simulink model "AFMss_"  (R2016b)
settings: Solver=ode4  StartTime=0.0  StopTime=trun  FixedStep=Ts  RelTol=1e-5  EnableMultiTasking=on
PreLoadFcn:
  | VSS_CONTROL_MODE=1;
  | VSS_LINEAR_CONTROL=Simulink.Variant('VSS_CONTROL_MODE==1');
  | VSS_MPC_CONTROL=Simulink.Variant('VSS_CONTROL_MODE == 2');
  | 
  | 
  | VSS_STATE_DIRECT=Simulink.Variant('VSS_STATE_MODE==1');
  | VSS_STATE_OBS=Simulink.Variant('VSS_STATE_MODE==2');
  | VSS_STATE_DIST_OBS=Simulink.Variant('VSS_STATE_MODE==3');
  | VSS_STATE_MODE=1;
values from neighbouring files (symbols this model uses):
  dist = 1    [explore_ss_loops_distest.m]    (also in explore_ss_loops_distest_AFM.m = 0; explore_ss_loops_distest_delta.m = 0)
  K_lqr = dlqr(sys.a, sys.b, Q, R, S)    [explore_ss_loops_distest.m]    (also in explore_ss_loops_distest_AFM.m; explore_ss_loops_distest_delta.m = dlqr(sys_recyc.a, sys_recyc.b, Q, R, S))
  L = dlqr(sys.a', sys.c', Q, R)'    [explore_ss_loops.m]
  Nbar = SSTools.getNbar(sys, K)    [explore_ss_loops.m]    (also in explore_ss_loops_distest.m = SSTools.getNbar(sys, K_lqr); explore_ss_loops_distest_AFM.m = SSTools.getNbar(sys, K_lqr); explore_ss_loops_distest_delta.m = SSTools.getNbar(sys_recyc, K_lqr))
  PLANT = sys    [explore_ss_loops_distest.m]    (also in explore_ss_loops_distest_AFM.m; explore_ss_loops_distest_delta.m)
  ref = 0    [explore_ss_loops_distest.m]    (also in explore_ss_loops_distest_AFM.m = 1; explore_ss_loops_distest_delta.m = 1)
  sys_obs = sys    [explore_ss_loops_distest_AFM.m]    (also in explore_ss_loops_distest_delta.m)
  Ts = 0.01    [explore_ss_loops.m]    (also in explore_ss_loops_GM_delta.m = plants.SYS.Ts; explore_ss_loops_distest.m; explore_ss_loops_distest_AFM.m = sys.Ts; explore_ss_loops_distest_delta.m = sys.Ts)
  x0 = PLANT.b*0    [explore_ss_loops_distest.m]    (also in explore_ss_loops_distest_AFM.m; explore_ss_loops_distest_delta.m)
  x0_obs = sys_obs.b*0    [explore_ss_loops_distest.m]    (also in explore_ss_loops_distest_AFM.m; explore_ss_loops_distest_delta.m)
settings Model: Creator=arnold  LastModifiedBy=arnold
settings DataIOCC: SaveFormat=Array  SaveOutput=off  SaveState=on  InspectSignalLogs=on  TimeSaveName=tout_ptos
settings OptimizationCC: LifeSpan=inf
settings DebuggingCC: SolverPrmCheckMsg=warning  SFUnexpectedBacktrackingDiag=warning  SFNoUnconditionalDefaultTransitionDiag=warning  SFExecutionAtInitializationDiag=none
settings HardwareCC: ProdBitPerPointer=32  ProdBitPerSizeT=32  ProdBitPerPtrDiffT=32  ProdLargestAtomicFloat=None  ProdIntDivRoundTo=Undefined  ProdEndianess=Unspecified  ProdWordSize=32  ProdHWDeviceType=32-bit Generic
settings ModelReferenceCC: PropagateSignalLabelsOutOfModel=off
settings GRTTargetCC: TargetLangStandard=C89/C90 (ANSI)  GeneratePreprocessorConditionals=Disable all
settings ConfigComp: CovMetricSettings=dw  CovHtmlReporting=on  CovSaveCumulativeToWorkspaceVar=on  CovSaveSingleToWorkspaceVar=on  CovExternalEMLEnable=off  CovSFcnEnable=off

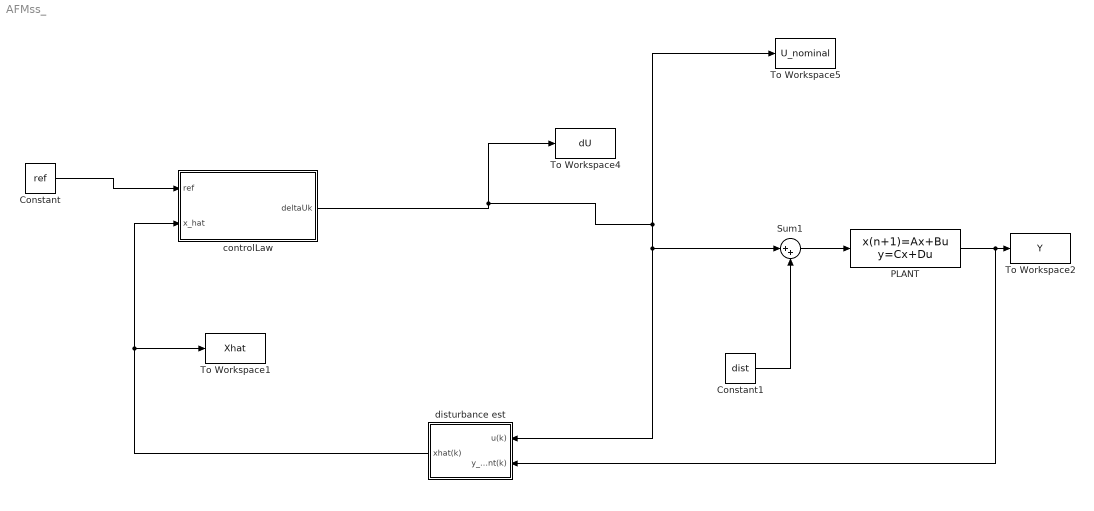
== system AFMss_ ==
  Constant : Constant  Value=ref
  Constant1 : Constant  Value=dist
  PLANT : DiscreteStateSpace  A=PLANT.a  B=PLANT.b  C=PLANT.c  D=zeros(size(PLANT.c,1),1)  X0=x0  SampleTime=Ts
  Sum1 : Sum  Inputs=|++
  To Workspace1 : ToWorkspace  VariableName=Xhat  SaveFormat=Timeseries  SampleTime=-1
      settings: Save2DSignal=2-D array (concatenate along first dimension)
  To Workspace2 : ToWorkspace  VariableName=Y  SaveFormat=Timeseries  SampleTime=-1
      settings: Save2DSignal=2-D array (concatenate along first dimension)
  To Workspace4 : ToWorkspace  VariableName=dU  SaveFormat=Timeseries  SampleTime=-1
      settings: Save2DSignal=2-D array (concatenate along first dimension)
  To Workspace5 : ToWorkspace  VariableName=U_nominal  SaveFormat=Timeseries  SampleTime=-1
      settings: Save2DSignal=2-D array (concatenate along first dimension)
  controlLaw : Subsystem
  disturbance est : Subsystem  VariantControl=VSS_STATE_DIST_OBS
  wires:
  PLANT/1 -> disturbance est/2(y_plant(k)), To Workspace2/1
  Sum1/1 -> PLANT/1
  controlLaw/1(deltaUk) -> Sum1/1, disturbance est/1(u(k)), To Workspace5/1, To Workspace4/1
  Constant/1 -> controlLaw/1(ref)
  disturbance est/1(xhat(k)) -> To Workspace1/1, controlLaw/2(x_hat)
  Constant1/1 -> Sum1/2

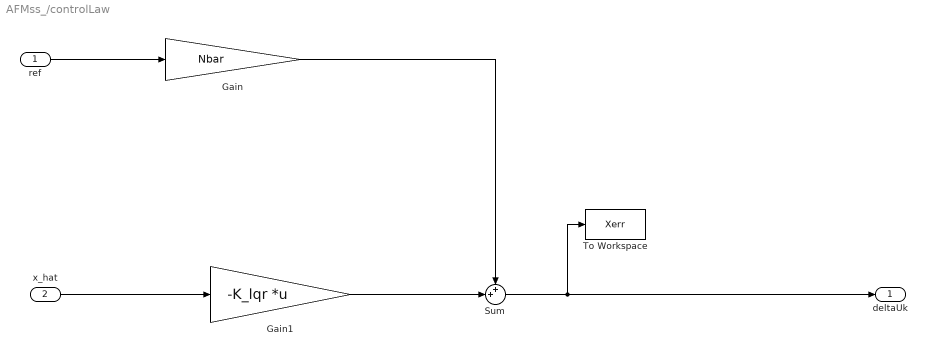
== system AFMss_/controlLaw ==
  ref : Inport
  x_hat : Inport  Port=2
  Gain : Gain  Gain=Nbar
  Gain1 : Gain  Gain=-K_lqr  Multiplication=Matrix(K*u)
  Sum : Sum  Inputs=++|
  To Workspace : ToWorkspace  VariableName=Xerr  SaveFormat=Timeseries  SampleTime=-1
  deltaUk : Outport
  wires:
  Sum/1 -> deltaUk/1, To Workspace/1
  x_hat/1 -> Gain1/1
  Gain/1 -> Sum/1
  ref/1 -> Gain/1
  Gain1/1 -> Sum/2

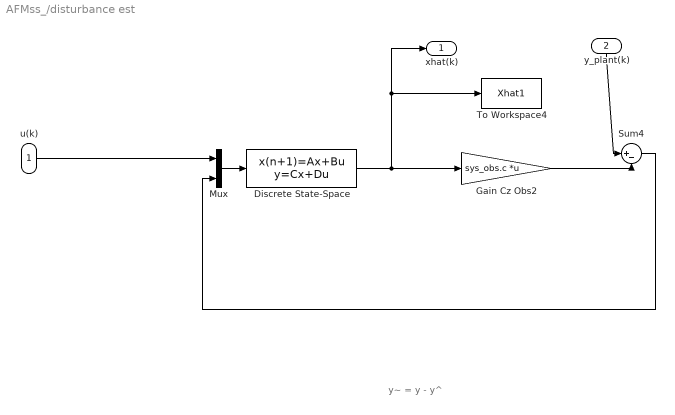
== system AFMss_/disturbance est ==
  note: y~ = y - y^
  u(k) : Inport
  y_plant(k) : Inport  Port=2
  Discrete State-Space : DiscreteStateSpace  A=sys_obs.a  B=[sys_obs.b, L]  C=eye(length(sys_obs.b))  D=zeros(length(sys_obs.b), 2)  X0=x0_obs  SampleTime=Ts
  Gain Cz Obs2 : Gain  Gain=sys_obs.c  Multiplication=Matrix(K*u)
  Mux : Mux  Inputs=2
  Sum4 : Sum  Inputs=|+-
  To Workspace4 : ToWorkspace  VariableName=Xhat1  SaveFormat=Timeseries  SampleTime=-1
      settings: Save2DSignal=2-D array (concatenate along first dimension)
  xhat(k) : Outport
  wires:
  Sum4/1 -> Mux/2
  u(k)/1 -> Mux/1
  Mux/1 -> Discrete State-Space/1
  Discrete State-Space/1 -> Gain Cz Obs2/1, To Workspace4/1, xhat(k)/1
  Gain Cz Obs2/1 -> Sum4/2
  y_plant(k)/1 -> Sum4/1
